simulink model "Project_Model_simulink_versionSignalBuilder_7_7_Harness"  (R2021a)
settings: Solver=FixedStepDiscrete  StartTime=0.0  StopTime=10  FixedStep=0.2  RelTol=1e-3
undefined symbols (not defined in the file or in its folder): sigbuilder_block
settings Model: Creator=A  LastModifiedBy=A
settings SolverCC: AlgebraicLoopSolver=TrustRegion
settings OptimizationCC: DefaultParameterBehavior=Inlined  EnhancedBackFolding=on  PassReuseOutputArgsAs=Individual arguments  ZeroExternalMemoryAtStartup=off  ZeroInternalMemoryAtStartup=off  OptimizeBlockOrder=speed  DifferentSizesBufferReuse=on  OptimizationCustomize=off  EfficientTunableParamExpr=on
settings DebuggingCC: ParameterPrecisionLossMsg=none  ParameterTunabilityLossMsg=error
settings SFSimCC: MATLABDynamicMemAlloc=off
settings RTWCC: SystemTargetFile=ert.tlc  TemplateMakefile=ert_default_tmf  GenerateReport=on  LaunchReport=on
settings CodeAppCC: ForceParamTrailComments=on  IgnoreCustomStorageClasses=off  OperatorAnnotations=on  SimulinkDataObjDesc=on  SFDataObjDesc=on  InsertBlockDesc=on
settings ERTTargetCC: TargetLangStandard=C99 (ISO)  GenerateSampleERTMain=on  InlinedParameterPlacement=NonHierarchical  ERTCustomFileTemplate=example_file_process.tlc
settings ConfigComp: CovEnable=on  RecordCoverage=on  CovMetricSettings=dzwe  CovHTMLOptions=-sRT=1 -sVT=1 -aTS=1 -agT=1 -bRG=1 -bTC=1 -hTR=0 -nFC=0 -nFD=1 -scm=1 -bcm=1 -xEv=0 -xEM=0 -req=1  CovSaveSingleToWorkspaceVar=on  CovCumulativeReport=on  CovModelRefEnable=on

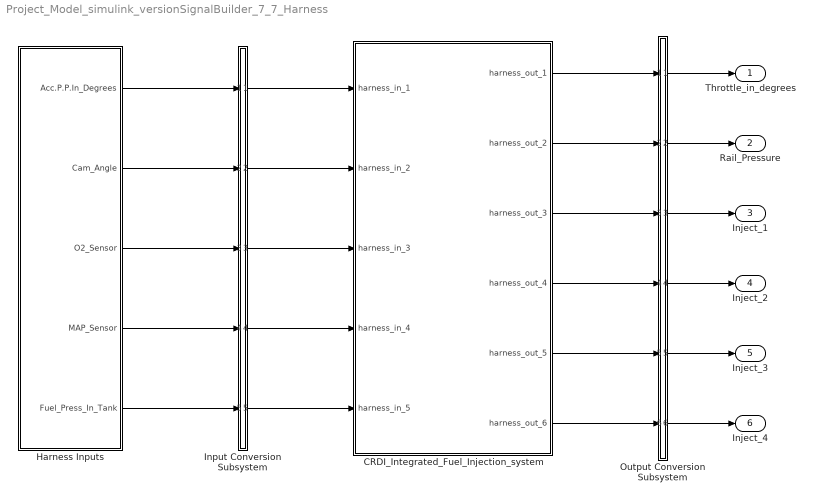
== system Project_Model_simulink_versionSignalBuilder_7_7_Harness ==
  CRDI_Integrated_Fuel_Injection_system : Subsystem  Tag=__SL_testing_harness_stub_
  Harness Inputs : Subsystem  Tag=STV Subsys  LoadFcn=sigbuilder_block('load',[50 50 520 400 ]);  StartFcn=sigbuilder_block('start');  StopFcn=sigbuilder_block('stop');  ClipboardFcn=sigbuilder_block('clipboard');  mask(Sigbuilder block){tuvar=[0:10]}
      mask init:
      | if ~strcmp(get_param(bdroot(gcb),'SimulationStatus'),'stopped'),tuvar = sigbuilder_block('maskInit'); end
      settings: CopyFcn=sigbuilder_block('copy');  DeleteFcn=sigbuilder_block('delete');  ModelCloseFcn=sigbuilder_block('modelClose');  PreSaveFcn=sigbuilder_block('preSave');  PauseFcn=sigbuilder_block('pause');  ContinueFcn=sigbuilder_block('continue');  NameChangeFcn=sigbuilder_block('namechange');  OpenFcn=sigbuilder_block('open',[50 50 520 400 ]);  CloseFcn=sigbuilder_block('close');
      mask Display: plot(0, 0, 100, 100,[2, 2, 32, 32, 2], [68, 8, 8, 68, 68],[32, 2], [38, 38], [32, 19, 2],[53, 60, 44], [32, 17, 17, 2],[16, 16, 31, 31]);txt = getActiveGroup(gcbh);text(2, 100, txt,'verticalAlignment', 'top');
  Input Conversion Subsystem : Subsystem  Tag=__SLT_ICS__  Description=|
      | Signal spec.
      | and routing
      settings: AttributesFormatString=%<Description>
  Output Conversion Subsystem : Subsystem  Tag=__SLT_OCS__  Description=|
      | Signal spec.
      | and routing
      settings: AttributesFormatString=%<Description>
  Throttle_in_degrees : Outport
  Rail_Pressure : Outport  Port=2
  Inject_1 : Outport  Port=3
  Inject_2 : Outport  Port=4
  Inject_3 : Outport  Port=5
  Inject_4 : Outport  Port=6
  wires:
  Harness Inputs/1(Acc.P.P.In_Degrees) -> Input Conversion Subsystem/1(Inport_1)
  Harness Inputs/2(Cam_Angle) -> Input Conversion Subsystem/2(Inport_2)
  Harness Inputs/3(O2_Sensor) -> Input Conversion Subsystem/3(Inport_3)
  Harness Inputs/4(MAP_Sensor) -> Input Conversion Subsystem/4(Inport_4)
  Harness Inputs/5(Fuel_Press_In_Tank) -> Input Conversion Subsystem/5(Inport_5)
  Output Conversion Subsystem/1(Outport_1) -> Throttle_in_degrees/1
  Output Conversion Subsystem/2(Outport_2) -> Rail_Pressure/1
  Output Conversion Subsystem/3(Outport_3) -> Inject_1/1
  Output Conversion Subsystem/4(Outport_4) -> Inject_2/1
  Output Conversion Subsystem/5(Outport_5) -> Inject_3/1
  Output Conversion Subsystem/6(Outport_6) -> Inject_4/1
  Input Conversion Subsystem/1(Outport_1) -> CRDI_Integrated_Fuel_Injection_system/1(harness_in_1)
  Input Conversion Subsystem/2(Outport_2) -> CRDI_Integrated_Fuel_Injection_system/2(harness_in_2)
  Input Conversion Subsystem/3(Outport_3) -> CRDI_Integrated_Fuel_Injection_system/3(harness_in_3)
  Input Conversion Subsystem/4(Outport_4) -> CRDI_Integrated_Fuel_Injection_system/4(harness_in_4)
  Input Conversion Subsystem/5(Outport_5) -> CRDI_Integrated_Fuel_Injection_system/5(harness_in_5)
  CRDI_Integrated_Fuel_Injection_system/1(harness_out_1) -> Output Conversion Subsystem/1(Inport_1)
  CRDI_Integrated_Fuel_Injection_system/2(harness_out_2) -> Output Conversion Subsystem/2(Inport_2)
  CRDI_Integrated_Fuel_Injection_system/3(harness_out_3) -> Output Conversion Subsystem/3(Inport_3)
  CRDI_Integrated_Fuel_Injection_system/4(harness_out_4) -> Output Conversion Subsystem/4(Inport_4)
  CRDI_Integrated_Fuel_Injection_system/5(harness_out_5) -> Output Conversion Subsystem/5(Inport_5)
  CRDI_Integrated_Fuel_Injection_system/6(harness_out_6) -> Output Conversion Subsystem/6(Inport_6)

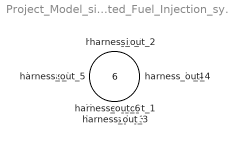
== system Project_Model_simulink_versionSignalBuilder_7_7_Harness/CRDI_Integrated_Fuel_Injection_system ==
  harness_in_1 : Inport
  harness_in_2 : Inport  Port=2
  harness_in_3 : Inport  Port=3
  harness_in_4 : Inport  Port=4
  harness_in_5 : Inport  Port=5
  harness_out_1 : Outport
  harness_out_2 : Outport  Port=2
  harness_out_3 : Outport  Port=3
  harness_out_4 : Outport  Port=4
  harness_out_5 : Outport  Port=5
  harness_out_6 : Outport  Port=6

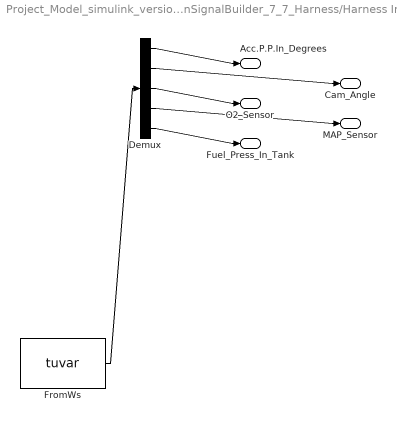
== system Project_Model_simulink_versionSignalBuilder_7_7_Harness/Harness Inputs ==
  Demux : Demux  Tag=STV Demux  Outputs=5
  FromWs : FromWorkspace  Tag=STV FromWs  VariableName=tuvar
      SigBuilderData=|
      | dataSet.timeRange = [0 4]
      | dataSet.name = 'Sheet1'
      | sbobj.Name = 'Signal Builder'
      | sbobj.Groups.Name = 'Sheet1'
      | sbobj.Groups.Signals(1).Name = 'Acc.P.P.In_Degrees'
      | sbobj.Groups.Signals(1).XData = [0 0.2 0.4 0.6 0.8 1 1.2 1.4 1.6 1.8 2 2.2 2.4 2.6 2.8 3 3.2 3.4 3.6 3.8 4]
      | sbobj.Groups.Signals(1).YData = [0 10 12 14 16 18 20 22 24 26 28 30 52 56 60 66 70 78 82 86 90]
      | sbobj.Groups.Signals(2).Name = 'Cam_Angle'
      | sbobj.Groups.Signals(2).XData = [0 0.2 0.4 0.6 0.8 1 1.2 1.4 1.6 1.8 2 2.2 2.4 2.6 2.8 3 3.2 3.4 3.6 3.8 4]
      | sbobj.Groups.Signals(2).YData = [177.5 179 180 183 184.5 222 224 225 229 267 269 270 272 274.5 313 314 315 319.2 340 345 350]
      | sbobj.Groups.Signals(3).Name = 'O2_Sensor'
      | sbobj.Groups.Signals(3).XData = [0 0.2 0.4 0.6 0.8 1 1.2 1.4 1.6 1.8 2 2.2 2.4 2.6 2.8 3 3.2 3.4 3.6 3.8 4]
      | sbobj.Groups.Signals(3).YData = [0.6 0.65 0.85 0.45 0.46 0.65 0.34 0.36 0.55 0.65 0.64 0.67 0.78 0.54 0.44 0.6 0.73 0.3 0.25 0.2 0.26]
      | sbobj.Groups.Signals(4).Name = 'MAP_Sensor'
      | sbobj.Groups.Signals(4).XData = [0 0.2 0.4 0.6 0.8 1 1.2 1.4 1.6 1.8 2 2.2 2.4 2.6 2.8 3 3.2 3.4 3.6 3.8 4]
      | sbobj.Groups.Signals(4).YData = [24 24.15 24.3 24.45 24.5 24.75 24.9 25.05 25.2 25.35 25.5 25.5 27.3 27.6 27.9 28.1 28.65 29.25 29.55 29.85 30]
      | sbobj.Groups.Signals(5).Name = 'Fuel_Press_In_Tank'
      | sbobj.Groups.Signals(5).XData = [0 0.2 0.4 0.6 0.8 1 1.2 1.4 1.6 1.8 2 2.2 2.4 2.6 2.8 3 3.2 3.4 3.6 3.8 4]
      | sbobj.Groups.Signals(5).YData = [1 1 1 1 1 1 1 1 1 1 1 1 1 1 1 1 1 1 1 1 1]
      | sbobj.Groups.TimeRange = [0 4]
  Acc.P.P.In_Degrees : Outport  Tag=STV Outport
  Cam_Angle : Outport  Tag=STV Outport  Port=2
  O2_Sensor : Outport  Tag=STV Outport  Port=3
  MAP_Sensor : Outport  Tag=STV Outport  Port=4
  Fuel_Press_In_Tank : Outport  Tag=STV Outport  Port=5
  wires:
  FromWs/1 -> Demux/1
  Demux/1 -> Acc.P.P.In_Degrees/1
  Demux/2 -> Cam_Angle/1
  Demux/3 -> O2_Sensor/1
  Demux/4 -> MAP_Sensor/1
  Demux/5 -> Fuel_Press_In_Tank/1

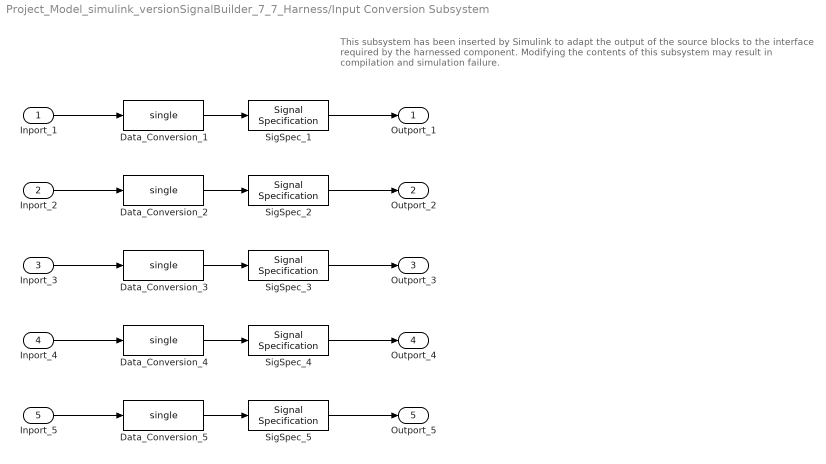
== system Project_Model_simulink_versionSignalBuilder_7_7_Harness/Input Conversion Subsystem ==
  note: This subsystem has been inserted by Simulink to adapt the output of the source blocks to the interface required by the harnessed component.
      |  Modifying the contents of this subsystem may result in compilation and simulation failure.
  Inport_1 : Inport
  Inport_2 : Inport  Port=2
  Inport_3 : Inport  Port=3
  Inport_4 : Inport  Port=4
  Inport_5 : Inport  Port=5
  Data_Conversion_{1..5} (5 alike) : DataTypeConversion  OutDataTypeStr=single  SaturateOnIntegerOverflow=on  RndMeth=Zero
  SigSpec_{1..5} (5 alike) : SignalSpecification  OutDataTypeStr=single  Dimensions=[1]  SampleTime=[0, 0]
  Outport_1 : Outport
  Outport_2 : Outport  Port=2
  Outport_3 : Outport  Port=3
  Outport_4 : Outport  Port=4
  Outport_5 : Outport  Port=5
  wires:
  SigSpec_1/1 -> Outport_1/1
  Data_Conversion_1/1 -> SigSpec_1/1
  Inport_1/1 -> Data_Conversion_1/1
  SigSpec_2/1 -> Outport_2/1
  Data_Conversion_2/1 -> SigSpec_2/1
  Inport_2/1 -> Data_Conversion_2/1
  SigSpec_3/1 -> Outport_3/1
  Data_Conversion_3/1 -> SigSpec_3/1
  Inport_3/1 -> Data_Conversion_3/1
  SigSpec_4/1 -> Outport_4/1
  Data_Conversion_4/1 -> SigSpec_4/1
  Inport_4/1 -> Data_Conversion_4/1
  SigSpec_5/1 -> Outport_5/1
  Data_Conversion_5/1 -> SigSpec_5/1
  Inport_5/1 -> Data_Conversion_5/1

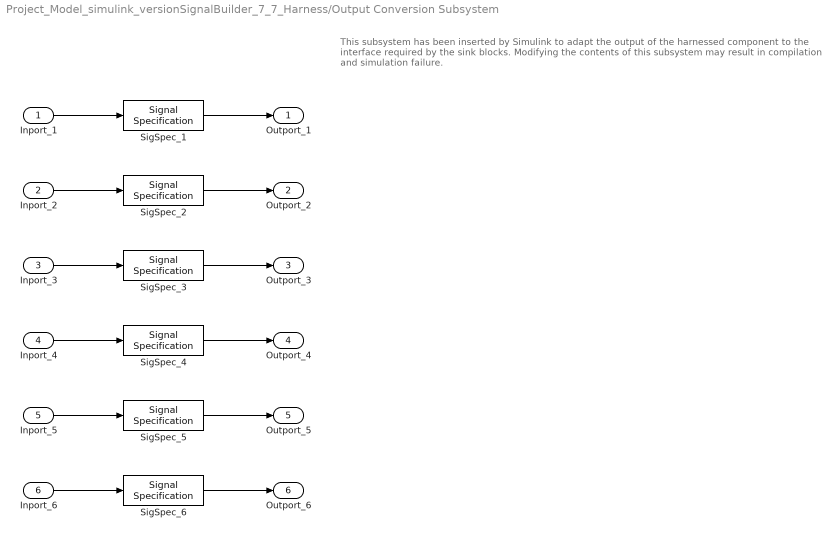
== system Project_Model_simulink_versionSignalBuilder_7_7_Harness/Output Conversion Subsystem ==
  note: This subsystem has been inserted by Simulink to adapt the output of the harnessed component to the interface required by the sink blocks.
      |  Modifying the contents of this subsystem may result in compilation and simulation failure.
  Inport_1 : Inport
  Inport_2 : Inport  Port=2
  Inport_3 : Inport  Port=3
  Inport_4 : Inport  Port=4
  Inport_5 : Inport  Port=5
  Inport_6 : Inport  Port=6
  SigSpec_{1..6} (6 alike) : SignalSpecification  OutDataTypeStr=single  Dimensions=[1]
  Outport_1 : Outport
  Outport_2 : Outport  Port=2
  Outport_3 : Outport  Port=3
  Outport_4 : Outport  Port=4
  Outport_5 : Outport  Port=5
  Outport_6 : Outport  Port=6
  wires:
  Inport_1/1 -> SigSpec_1/1
  SigSpec_1/1 -> Outport_1/1
  Inport_2/1 -> SigSpec_2/1
  SigSpec_2/1 -> Outport_2/1
  Inport_3/1 -> SigSpec_3/1
  SigSpec_3/1 -> Outport_3/1
  Inport_4/1 -> SigSpec_4/1
  SigSpec_4/1 -> Outport_4/1
  Inport_5/1 -> SigSpec_5/1
  SigSpec_5/1 -> Outport_5/1
  Inport_6/1 -> SigSpec_6/1
  SigSpec_6/1 -> Outport_6/1
